simulink model "VSD_Motor_20kW"  (Simulink 9.3)
settings: Solver=ode23t  StartTime=0.0  StopTime=2  FixedStep=1e-5  MaxStep=1e-5  MinStep=1e-7  RelTol=1e-6  AbsTol=1e-6  EnableMultiTasking=on
libraries: powerlib x24, powerlib_extras x6, simulink x2
(part 1 of 2)
settings Model: Creator=Jiang  LastModifiedBy=Dominion
settings SolverCC: AutoScaleAbsTol=off
settings DataIOCC: LimitDataPoints=on
settings OptimizationCC: ExpressionDepthLimit=2147483647  InitFltsAndDblsToZero=on
settings DebuggingCC: SaveWithParameterizedLinksMsg=none  SignalResolutionControl=TryResolveAllWithWarning  SolverPrmCheckMsg=warning  MultiTaskDSMMsg=warning  MultiTaskCondExecSysMsg=none  StateNameClashWarn=warning
settings SFSimCC: SimUseLocalCustomCode=on
settings RTWCC: RTWUseLocalCustomCode=on
settings GRTTargetCC: TargetFcnLib=ansi_tfl_tmw.mat
settings ConfigComp: CovExternalEMLEnable=on

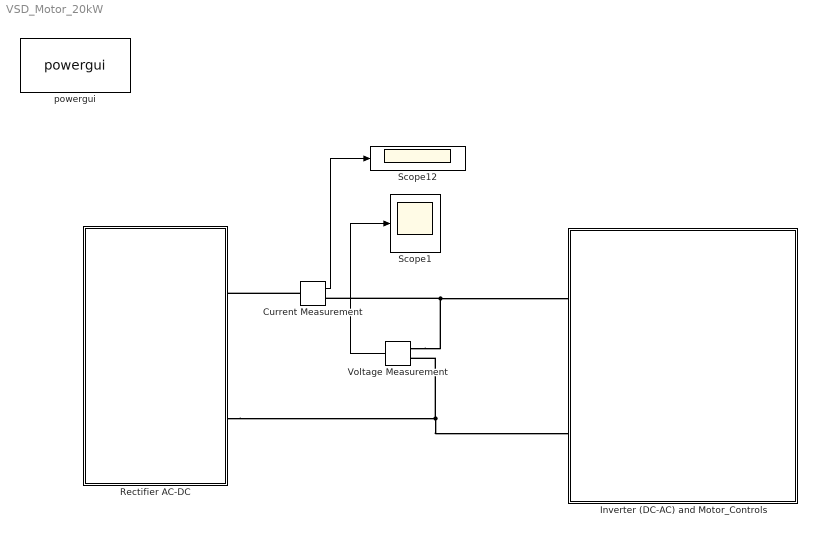
== system VSD_Motor_20kW ==
  Current Measurement : powerlib/Measurements/Current Measurement  PhasorSimulation=off  OutputType=Complex  PSBequivalent=0
      settings: SourceProductName=Simscape Electrical
  Inverter (DC-AC) and Motor_Controls : Subsystem
  Rectifier AC-DC : Subsystem
  Scope1 : Scope
  Scope12 : Scope
  Voltage Measurement : powerlib/Measurements/Voltage Measurement  PhasorSimulation=off  OutputType=Complex  PSBequivalent=0
      settings: SourceProductName=Simscape Electrical
  powergui : powerlib/powergui  SimulationMode=Discrete  SampleTime=2e-6  frequency=60  Iterations=50  frequencyindice=0  Pbase=100e6  ErrMax=1e-4  UnitsV=kV  UnitsW=MW  buscounter=0  FunctionMessages=off  echomessages=off  EnableUseOfTLC=off  CurrentSourceSwitches=off  DisableSnubberDevices=off  DisableRonSwitches=off  DisableVfSwitches=off  DisplayEquations=off  AutomaticDiscreteSolvers=off  SolverType=Tustin/Backward Euler (TBE)  Interpol=off  ExternalGateDelay=off  methode=off  Ts=0  x0status=blocks  SPID=off  SwTol=0  HookPort=off  NonlinearTolerance=0  nMaxIteration=15  ContinueOnMaxIteration=off  RestoreLinks=warning  ResistiveCurrentMeasurement=off  Frange=[0:2:500]  Ylog=off  Xlog=on  ShowGrid=off  save=off  variable=ZData  structure=0  ZoomFFT=on  StartTime=0.0  cycles=1  DisplayStyle=1  fundamental=60  FreqAxis=off  MaxFrequency=1000  frequencyindicesteady=1  RmsSteady=1  display=off
      settings: SourceProductName=Simscape Electrical
  wires:
  Voltage Measurement/1 -> Scope1/1
  Current Measurement/1 -> Scope12/1
  connections:
  Current Measurement/LConn1 -- Rectifier AC-DC/RConn1
  Voltage Measurement/LConn1 -- Current Measurement/RConn1 -- Inverter (DC-AC) and Motor_Controls/LConn1
  Rectifier AC-DC/RConn2 -- Voltage Measurement/LConn2 -- Inverter (DC-AC) and Motor_Controls/LConn2

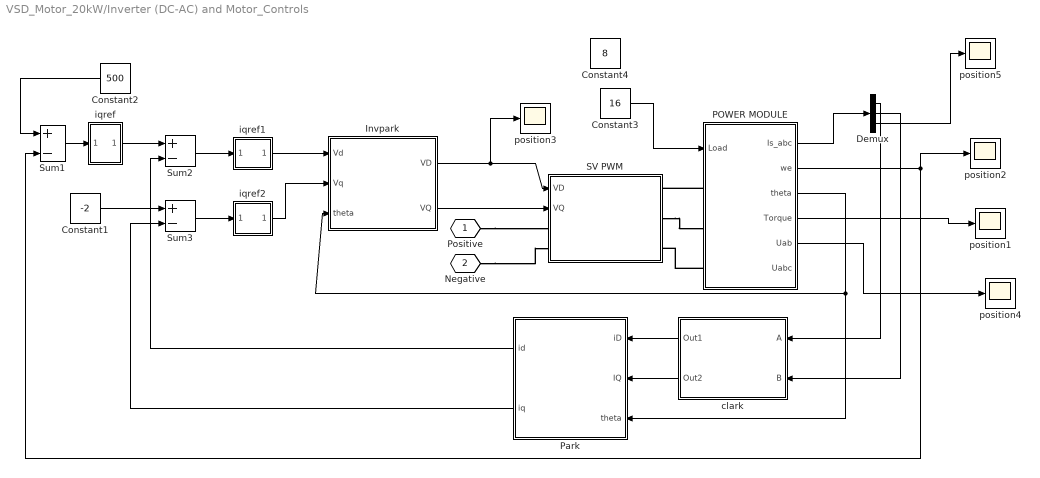
== system VSD_Motor_20kW/Inverter (DC-AC) and Motor_Controls ==
  Constant1 : Constant  Value=-2
  Constant2 : Constant  Value=500
  Constant3 : Constant  Value=16
  Constant4 : Constant  Value=8
  Demux : Demux  Outputs=3
  Invpark : Subsystem
  POWER MODULE : Subsystem
  Park : Subsystem
  SV PWM : Subsystem
  Sum1 : Sum  Inputs=+-  SaturateOnIntegerOverflow=on  InputSameDT=on  OutDataTypeStr=Inherit: Same as first input
  Sum2 : Sum  Inputs=+-  SaturateOnIntegerOverflow=on  InputSameDT=on  OutDataTypeStr=Inherit: Same as first input
  Sum3 : Sum  Inputs=+-  SaturateOnIntegerOverflow=on  InputSameDT=on  OutDataTypeStr=Inherit: Same as first input
  clark : Subsystem
  iqref : Subsystem  mask(PI Controller){I=20, P=0.2, sat=[-30,30]}
      mask prompts: I "Integral"; P "Proportional:"; sat "Minimum and maximum outputs:"
      mask init:
      | min=sat(1);max=sat(2);
      mask Display: disp('PI')
  iqref1 : Subsystem  mask(PI Controller){I=100, P=30, sat=[-400,400]}
      mask prompts: I "Integral"; P "Proportional:"; sat "Minimum and maximum outputs:"
      mask init:
      | min=sat(1);max=sat(2);
      mask Display: disp('PI')
  iqref2 : Subsystem  mask(PI Controller){I=100, P=30, sat=[-400,400]}
      mask prompts: I "Integral"; P "Proportional:"; sat "Minimum and maximum outputs:"
      mask init:
      | min=sat(1);max=sat(2);
      mask Display: disp('PI')
  position{1..5} (5 alike) : Scope
  Positive : PMIOPort  Tag=PMCPort  Side=Left
  Negative : PMIOPort  Tag=PMCPort  Port=2  Side=Left
  wires:
  Invpark/1(VD) -> SV PWM/1(VD), position3/1
  Invpark/2(VQ) -> SV PWM/2(VQ)
  Constant3/1 -> POWER MODULE/1(Load)
  POWER MODULE/1(Is_abc) -> Demux/1
  Demux/3 -> position5/1
  POWER MODULE/4(Torque) -> position1/1
  POWER MODULE/2(we) -> position2/1, Sum1/2
  Demux/1 -> clark/1(A)
  Demux/2 -> clark/2(B)
  clark/1(Out1) -> Park/1(iD)
  clark/2(Out2) -> Park/2(IQ)
  POWER MODULE/3(theta) -> Invpark/3(theta), Park/3(theta)
  Sum2/1 -> iqref1/1(In_1)
  Sum3/1 -> iqref2/1(In_1)
  Sum1/1 -> iqref/1(In_1)
  iqref2/1(Out_1) -> Invpark/2(Vq)
  iqref1/1(Out_1) -> Invpark/1(Vd)
  iqref/1(Out_1) -> Sum2/1
  Constant1/1 -> Sum3/1
  Constant2/1 -> Sum1/1
  Park/2(iq) -> Sum3/2
  Park/1(id) -> Sum2/2
  POWER MODULE/5(Uab) -> position4/1
  connections:
  POWER MODULE/LConn1 -- SV PWM/RConn1
  SV PWM/RConn2 -- POWER MODULE/LConn2
  POWER MODULE/LConn3 -- SV PWM/RConn3
  Negative/RConn1 -- SV PWM/LConn2
  Positive/RConn1 -- SV PWM/LConn1

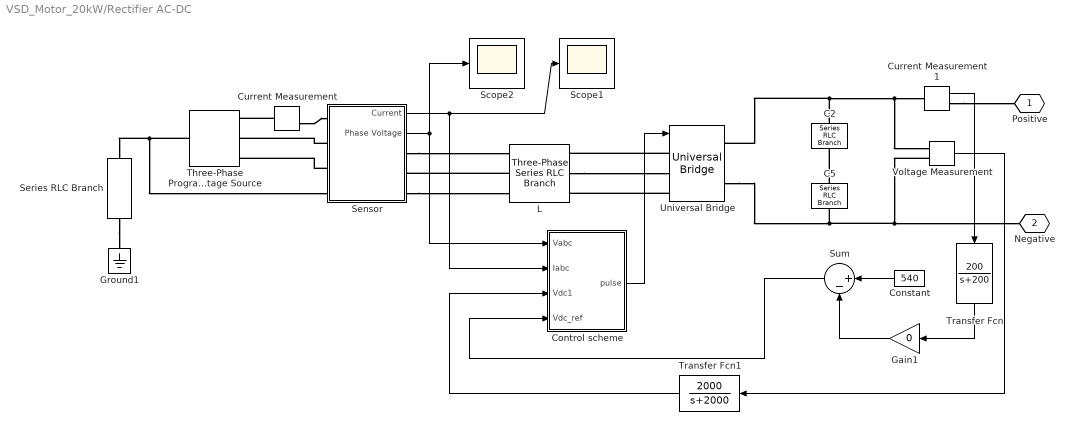
== system VSD_Motor_20kW/Rectifier AC-DC ==
  C2 : powerlib/Elements/Series RLC Branch  LConnTagsString=__new0  RConnTagsString=__new0  BranchType=C  Resistance=1.0  Inductance=1.0  SetiL0=off  InitialCurrent=0  Capacitance=6e-04  Setx0=on  InitialVoltage=100  Measurements=None
      settings: SourceProductName=Simscape Electrical
  C5 : powerlib/Elements/Series RLC Branch  LConnTagsString=__new0  RConnTagsString=__new0  BranchType=C  Resistance=1.0  Inductance=1.0  SetiL0=off  InitialCurrent=0  Capacitance=6e-04  Setx0=on  InitialVoltage=100  Measurements=None
      settings: SourceProductName=Simscape Electrical
  Constant : Constant  Value=540
  Control scheme : Subsystem
  Current Measurement : powerlib/Measurements/Current Measurement  PhasorSimulation=off  OutputType=Complex  PSBequivalent=0
      settings: SourceProductName=Simscape Electrical
  Current Measurement1 : powerlib/Measurements/Current Measurement  PhasorSimulation=off  OutputType=Complex  PSBequivalent=0
      settings: SourceProductName=Simscape Electrical
  Gain1 : Gain  Gain=0
  Ground1 : powerlib/Elements/Ground  LConnTagsString=a
      settings: SourceProductName=Simscape Electrical
  L : powerlib/Elements/Three-Phase Series RLC Branch  LConnTagsString=A|B|C  RConnTagsString=A|B|C  BranchType=RL  Resistance=0.0001  Inductance=3.5e-3  Capacitance=1.0  Measurements=None
      settings: SourceProductName=Simscape Electrical
  Scope1 : Scope
  Scope2 : Scope
  Sensor : Subsystem
  Series RLC Branch : powerlib/Elements/Series RLC Branch  LConnTagsString=__new0  RConnTagsString=__new0  BranchType=R  Resistance=1e5  Inductance=1e-3  SetiL0=off  InitialCurrent=0  Capacitance=1e-6  Setx0=off  InitialVoltage=0  Measurements=None
      settings: SourceProductName=Simscape Electrical
  Sum : Sum  Inputs=|+-  SaturateOnIntegerOverflow=on  InputSameDT=on  OutDataTypeStr=Inherit: Same as first input
  Three-Phase Programmable Voltage Source : powerlib/Electrical Sources/Three-Phase Programmable Voltage Source  PositiveSequence=[400 0 60]  VariationEntity=None  VariationType=Step  VariationTypeAlt=Step  VariationStep=0.5  VariationRate=10  VariationMagnitude=0.3  VariationFrequency=2  VariationTiming=[1 2]  VariationPhaseA=off  Amplitudes=[1 0.8 1.2 1.0]  TimeValues=[0 0.1 0.15 0.2]  HarmonicGeneration=off  HarmonicA=[3 0.2 -25 0]  HarmonicB=[2 0.15 35 2]  Timing="[0.05  3]"  BusType=swing  Pref=0  Qref=0  Qmin=-inf  Qmax=inf
      settings: SourceProductName=Simscape Electrical
  Transfer Fcn : TransferFcn  Numerator=[200]  Denominator=[1 200]
  Transfer Fcn1 : TransferFcn  Numerator=[2000]  Denominator=[1 2000]
  Universal Bridge : powerlib/Power Electronics/Universal Bridge  Arms=3  SnubberResistance=50000  SnubberCapacitance=1e-8  Device=MOSFET / Diodes  Ron=0.2e-4  Lon=0  ForwardVoltages="[  2 1  ]"  ForwardVoltage=0  GTOparameters=[ 10e-6 , 20e-6 ]  IGBTparameters=[ 1e-6 , 2e-6 ]  Measurements=None  Measurements_2=None  converterType=Rectifier
      settings: SourceProductName=Simscape Electrical
  Voltage Measurement : powerlib/Measurements/Voltage Measurement  PhasorSimulation=off  OutputType=Complex  PSBequivalent=0
      settings: SourceProductName=Simscape Electrical
  Positive : PMIOPort  Tag=PMCPort  Side=Right
  Negative : PMIOPort  Tag=PMCPort  Port=2  Side=Right
  wires:
  Voltage Measurement/1 -> Transfer Fcn1/1
  Control scheme/1(pulse) -> Universal Bridge/1
  Constant/1 -> Sum/1
  Gain1/1 -> Sum/2
  Sum/1 -> Control scheme/4(Vdc_ref)
  Sensor/1(Current) -> Control scheme/2(Iabc), Scope1/1
  Sensor/2(Phase Voltage) -> Control scheme/1(Vabc), Scope2/1
  Transfer Fcn/1 -> Gain1/1
  Transfer Fcn1/1 -> Control scheme/3(Vdc1)
  Current Measurement1/1 -> Transfer Fcn/1
  connections:
  L/LConn2 -- Sensor/RConn2
  Universal Bridge/LConn1 -- L/RConn1
  L/RConn2 -- Universal Bridge/LConn2
  Current Measurement/LConn1 -- Three-Phase Programmable Voltage Source/RConn1
  Sensor/RConn1 -- L/LConn1
  Universal Bridge/LConn3 -- L/RConn3
  Sensor/RConn3 -- L/LConn3
  Current Measurement/RConn1 -- Sensor/LConn1
  Sensor/LConn2 -- Three-Phase Programmable Voltage Source/RConn2
  Sensor/LConn3 -- Three-Phase Programmable Voltage Source/RConn3
  Universal Bridge/RConn1 -- C2/LConn1 -- Voltage Measurement/LConn1 -- Current Measurement1/LConn1
  Voltage Measurement/LConn2 -- Negative/RConn1 -- Universal Bridge/RConn2 -- C5/RConn1
  C5/LConn1 -- C2/RConn1
  Three-Phase Programmable Voltage Source/LConn1 -- Sensor/LConn4 -- Series RLC Branch/LConn1
  Current Measurement1/RConn1 -- Positive/RConn1
  Series RLC Branch/RConn1 -- Ground1/LConn1

== system VSD_Motor_20kW/Inverter (DC-AC) and Motor_Controls/Invpark ==
  Vd : Inport
  Vq : Inport  Port=2
  theta : Inport  Port=3
  Product{,1..3} (4 alike) : Product  RndMeth=Zero
  Sum2 : Sum  Inputs=|-+
  Sum3 : Sum  Inputs=|++
  Trigonometric Function : Trigonometry
  Trigonometric Function1 : Trigonometry  Operator=cos
  VD : Outport
  VQ : Outport  Port=2
  wires:
  Trigonometric Function1/1 -> Product/2, Product3/2
  Trigonometric Function/1 -> Product1/2, Product2/2
  Product1/1 -> Sum2/1
  Product/1 -> Sum2/2
  Sum2/1 -> VD/1
  Product2/1 -> Sum3/2
  Product3/1 -> Sum3/1
  Sum3/1 -> VQ/1
  theta/1 -> Trigonometric Function/1, Trigonometric Function1/1
  Vd/1 -> Product/1, Product2/1
  Vq/1 -> Product1/1, Product3/1

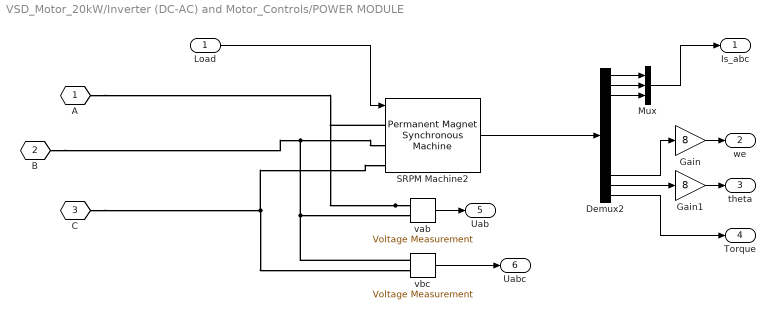
== system VSD_Motor_20kW/Inverter (DC-AC) and Motor_Controls/POWER MODULE ==
  Load : Inport
  Demux2 : Demux  Outputs=13
  Gain : Gain  Gain=8
  Gain1 : Gain  Gain=8
  Mux : Mux  Inputs=3
  SRPM Machine2 : powerlib/Machines/Permanent Magnet Synchronous Machine  NbPhases=3  FluxDistribution=Sinusoidal  RotorType=Round  MechanicalLoad=Torque Tm  PresetModel=No  ShowDetailedParameters=on  MeasurementBus=off  Resistance=0.7  Inductance=8.5e-3  dqInductances=[0.01 0.01]  La=0.000395  MachineConstant=Flux linkage established by magnets (V.s)  Flux=0.1  VoltageCst=145.1039  TorqueCst=1.2  Flat=120  Mechanical="[ 2e-4, 0,  8 ]"  PolePairs=4  InitialConditions=[0,0, 0,0]  InitialConditions5ph=[0 0 0 0 0 0]  TsPowergui=0  TsBlock=-1  RefAngle=90 degrees behind phase A axis (modified Park)
      settings: AttributesFormatString=\n
  vab : powerlib/Measurements/Voltage Measurement  Tag=PoWeRsYsTeMmEaSuReMeNt  PhasorSimulation=off  OutputType=Magnitude  PSBequivalent=0
      settings: SourceProductName=Simscape Electrical
  vbc : powerlib/Measurements/Voltage Measurement  Tag=PoWeRsYsTeMmEaSuReMeNt  PhasorSimulation=off  OutputType=Magnitude  PSBequivalent=0
      settings: SourceProductName=Simscape Electrical
  A : PMIOPort  Tag=PMCPort  Side=Left
  B : PMIOPort  Tag=PMCPort  Port=2  Side=Left
  C : PMIOPort  Tag=PMCPort  Port=3  Side=Left
  Is_abc : Outport
  we : Outport  Port=2
  theta : Outport  Port=3
  Torque : Outport  Port=4
  Uab : Outport  Port=5
  Uabc : Outport  Port=6
  wires:
  SRPM Machine2/1 -> Demux2/1
  Load/1 -> SRPM Machine2/1
  Demux2/1 -> Mux/1
  Demux2/2 -> Mux/2
  Demux2/3 -> Mux/3
  Mux/1 -> Is_abc/1
  Demux2/11 -> Gain/1
  Demux2/12 -> Gain1/1
  Demux2/13 -> Torque/1
  vab/1 -> Uab/1
  Gain/1 -> we/1
  Gain1/1 -> theta/1
  vbc/1 -> Uabc/1
  connections:
  vab/LConn1 -- A/RConn1 -- SRPM Machine2/LConn1
  vbc/LConn1 -- vab/LConn2 -- B/RConn1 -- SRPM Machine2/LConn2
  C/RConn1 -- SRPM Machine2/LConn3 -- vbc/LConn2

== system VSD_Motor_20kW/Inverter (DC-AC) and Motor_Controls/Park ==
  iD : Inport
  IQ : Inport  Port=2
  theta : Inport  Port=3
  Product{,1..3} (4 alike) : Product  RndMeth=Zero
  Sum1 : Sum  Inputs=|++
  Sum2 : Sum  Inputs=|+-
  Trigonometric Function : Trigonometry
  Trigonometric Function1 : Trigonometry  Operator=cos
  id : Outport
  iq : Outport  Port=2
  wires:
  theta/1 -> Trigonometric Function1/1, Trigonometric Function/1
  Trigonometric Function1/1 -> Product/2, Product3/2
  Trigonometric Function/1 -> Product1/2, Product2/2
  IQ/1 -> Product1/1, Product3/1
  iD/1 -> Product/1, Product2/1
  Product1/1 -> Sum1/1
  Product/1 -> Sum1/2
  Sum1/1 -> id/1
  Product2/1 -> Sum2/2
  Product3/1 -> Sum2/1
  Sum2/1 -> iq/1

== system VSD_Motor_20kW/Inverter (DC-AC) and Motor_Controls/SV PWM ==
  VD : Inport
  VQ : Inport  Port=2
  SVPWM : Subsystem  mask(SVPWM){Ts=1/2e4}
      mask prompts: Ts "switching frequency"
      mask help: two-level svpwm generator
  Universal Bridge1 : powerlib/Power Electronics/Universal Bridge  Arms=3  SnubberResistance=1e5  SnubberCapacitance=inf  Device=MOSFET / Diodes  Ron=1e-3  Lon=0  ForwardVoltages="[  0  0  ]"  ForwardVoltage=0  GTOparameters=[ 10e-6 , 20e-6 ]  IGBTparameters=[ 1e-6 , 2e-6 ]  Measurements=None  Measurements_2=None  converterType=Rectifier
      settings: SourceProductName=Simscape Electrical
  vdc : powerlib/Measurements/Voltage Measurement  Tag=PoWeRsYsTeMmEaSuReMeNt  PhasorSimulation=off  OutputType=Magnitude  PSBequivalent=0
      settings: SourceProductName=Simscape Electrical
  Positive : PMIOPort  Tag=PMCPort  Side=Left
  negative : PMIOPort  Tag=PMCPort  Port=2  Side=Left
  A : PMIOPort  Tag=PMCPort  Port=3  Side=Right
  B : PMIOPort  Tag=PMCPort  Port=4  Side=Right
  C : PMIOPort  Tag=PMCPort  Port=5  Side=Right
  wires:
  VD/1 -> SVPWM/2(Valf)
  VQ/1 -> SVPWM/3(Vbeta)
  SVPWM/1(Out1) -> Universal Bridge1/1
  vdc/1 -> SVPWM/1(Udc)
  connections:
  Positive/RConn1 -- Universal Bridge1/RConn1 -- vdc/LConn1
  negative/RConn1 -- Universal Bridge1/RConn2 -- vdc/LConn2
  C/RConn1 -- Universal Bridge1/LConn3
  B/RConn1 -- Universal Bridge1/LConn2
  A/RConn1 -- Universal Bridge1/LConn1

== system VSD_Motor_20kW/Inverter (DC-AC) and Motor_Controls/clark ==
  A : Inport
  B : Inport  Port=2
  Gain : Gain  Gain=3/2
  Gain1 : Gain  Gain=2/sqrt(3)
  Gain2 : Gain  Gain=1/sqrt(3)
  Gain3 : Gain  Gain=3/2
  Gain4 : Gain  Gain=sqrt(2/3)
  Gain5 : Gain  Gain=sqrt(2/3)
  Sum1 : Sum  Inputs=|++
  Out1 : Outport
  Out2 : Outport  Port=2
  wires:
  A/1 -> Gain2/1, Gain3/1
  B/1 -> Gain1/1
  Gain2/1 -> Sum1/1
  Gain1/1 -> Sum1/2
  Sum1/1 -> Gain/1
  Gain3/1 -> Gain4/1
  Gain/1 -> Gain5/1
  Gain4/1 -> Out1/1
  Gain5/1 -> Out2/1

== system VSD_Motor_20kW/Inverter (DC-AC) and Motor_Controls/iqref ==
  In_1 : Inport
  Integral : TransferFcn  Numerator=[I]  Denominator=[1 0]
  Proportional : Gain  Gain=P  SaturateOnIntegerOverflow=on  OutDataTypeStr=Inherit: Same as input  ParamDataTypeStr=Inherit: Same as input
  Saturation : Saturate  UpperLimit=max  LowerLimit=min
  Sum : Sum  SaturateOnIntegerOverflow=on  InputSameDT=on  OutDataTypeStr=Inherit: Same as first input
  Out_1 : Outport  InitialOutput=0
  wires:
  Integral/1 -> Sum/2
  In_1/1 -> Integral/1, Proportional/1
  Proportional/1 -> Sum/1
  Sum/1 -> Saturation/1
  Saturation/1 -> Out_1/1

== system VSD_Motor_20kW/Inverter (DC-AC) and Motor_Controls/iqref1 ==
  In_1 : Inport
  Integral : TransferFcn  Numerator=[I]  Denominator=[1 0]
  Proportional : Gain  Gain=P  SaturateOnIntegerOverflow=on  OutDataTypeStr=Inherit: Same as input  ParamDataTypeStr=Inherit: Same as input
  Saturation : Saturate  UpperLimit=max  LowerLimit=min
  Sum : Sum  SaturateOnIntegerOverflow=on  InputSameDT=on  OutDataTypeStr=Inherit: Same as first input
  Out_1 : Outport  InitialOutput=0
  wires:
  Integral/1 -> Sum/2
  In_1/1 -> Integral/1, Proportional/1
  Proportional/1 -> Sum/1
  Sum/1 -> Saturation/1
  Saturation/1 -> Out_1/1

== system VSD_Motor_20kW/Inverter (DC-AC) and Motor_Controls/iqref2 ==
  In_1 : Inport
  Integral : TransferFcn  Numerator=[I]  Denominator=[1 0]
  Proportional : Gain  Gain=P  SaturateOnIntegerOverflow=on  OutDataTypeStr=Inherit: Same as input  ParamDataTypeStr=Inherit: Same as input
  Saturation : Saturate  UpperLimit=max  LowerLimit=min
  Sum : Sum  SaturateOnIntegerOverflow=on  InputSameDT=on  OutDataTypeStr=Inherit: Same as first input
  Out_1 : Outport  InitialOutput=0
  wires:
  Integral/1 -> Sum/2
  In_1/1 -> Integral/1, Proportional/1
  Proportional/1 -> Sum/1
  Sum/1 -> Saturation/1
  Saturation/1 -> Out_1/1

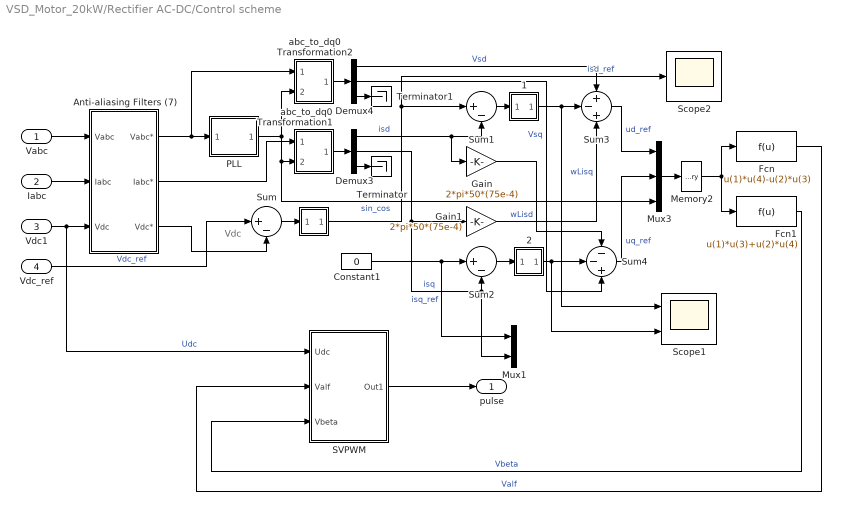
== system VSD_Motor_20kW/Rectifier AC-DC/Control scheme ==
  note: Vdc
  Vabc : Inport  PortDimensions=3
  Iabc : Inport  Port=2  PortDimensions=3
  Vdc1 : Inport  Port=3  PortDimensions=1
  Vdc_ref : Inport  Port=4  PortDimensions=1
  " " : Subsystem  mask(PI Controller){I=100, P=0.07, sat=[-200,200]}
      mask prompts: I "Integral"; P "Proportional:"; sat "Minimum and maximum outputs:"
      mask init:
      | min=sat(1);max=sat(2);
      mask Display: disp('PI')
  " 1" : Subsystem  mask(PI Controller){I=100, P=20, sat=[-1000*1.2, 1000*1.2]}
      mask prompts: I "Integral"; P "Proportional:"; sat "Minimum and maximum outputs:"
      mask init:
      | min=sat(1);max=sat(2);
      mask Display: disp('PI')
  " 2" : Subsystem  mask(PI Controller){I=100, P=20, sat=[-1000*1.2, 1000*1.2]}
      mask prompts: I "Integral"; P "Proportional:"; sat "Minimum and maximum outputs:"
      mask init:
      | min=sat(1);max=sat(2);
      mask Display: disp('PI')
  Anti-aliasing Filters (7) : Subsystem  mask(Anti-aliasing (2nd order lowpass)){Fc=750, Ts=-1}
      mask prompts: Fc "Cut-off frequency (Hz):"; Ts "Sample time:"
  Constant1 : Constant  Value=0
  Demux3 : Demux  Outputs=3
  Demux4 : Demux  Outputs=3
  Fcn : Fcn  Expr=u(1)*u(4)-u(2)*u(3)
  Fcn1 : Fcn  Expr=u(1)*u(3)+u(2)*u(4)
  Gain : Gain  Gain=2*pi*50*(75e-4)
  Gain1 : Gain  Gain=2*pi*50*(75e-4)
  Memory2 : Memory
  Mux1 : Mux  Inputs=2
  Mux3 : Mux  Inputs=3
  PLL : Subsystem
  SVPWM : Subsystem  mask(SVPWM){Ts=1/5e3}
      mask prompts: Ts "switching frequency"
      mask help: two-level svpwm generator
  Scope1 : Scope  NumInputPorts=2
  Scope2 : Scope
  Sum : Sum  Inputs=|+-  SaturateOnIntegerOverflow=on  InputSameDT=on  OutDataTypeStr=Inherit: Same as first input
  Sum1 : Sum  Inputs=|+-  SaturateOnIntegerOverflow=on  InputSameDT=on  OutDataTypeStr=Inherit: Same as first input
  Sum2 : Sum  Inputs=|+-  SaturateOnIntegerOverflow=on  InputSameDT=on  OutDataTypeStr=Inherit: Same as first input
  Sum3 : Sum  Inputs=+-+  SaturateOnIntegerOverflow=on  InputSameDT=on  OutDataTypeStr=Inherit: Same as first input
  Sum4 : Sum  Inputs=--+  SaturateOnIntegerOverflow=on  InputSameDT=on  OutDataTypeStr=Inherit: Same as first input
  Terminator : Terminator
  Terminator1 : Terminator
  abc_to_dq0 Transformation1 : Subsystem  mask(abc to dq0 Transformation){}
      mask help:
      | This block performs the  abc to dq0 transformation on a set of three-phase signals. It computes the direct axis Vd, quadratic axis Vq, and zero sequence V0 quantities in a two axis rotating reference frame according to the following transformation:
      |
      | Vd = 2/3*[Va*sin(wt)  + Vb*sin(wt-2pi/3)  +  Vc*sin(wt+2pi/3)]
      | Vq = 2/3*[Va*cos(wt) + Vb*cos(wt-2pi/3) + Vc*cos(wt+2pi/3)]
      | V0 = 1/3*[Va +  Vb  +  Vc ]
      |
      | where w=  rotation speed (rad/s) of the rotating frame.
      |
      | This transformation is commonly used in three-phase electric machine models where it is known as the Park transformation.
      mask Help: web(psbhelp);
  abc_to_dq0 Transformation2 : Subsystem  mask(abc to dq0 Transformation){}
      mask help:
      | This block performs the  abc to dq0 transformation on a set of three-phase signals. It computes the direct axis Vd, quadratic axis Vq, and zero sequence V0 quantities in a two axis rotating reference frame according to the following transformation:
      |
      | Vd = 2/3*[Va*sin(wt)  + Vb*sin(wt-2pi/3)  +  Vc*sin(wt+2pi/3)]
      | Vq = 2/3*[Va*cos(wt) + Vb*cos(wt-2pi/3) + Vc*cos(wt+2pi/3)]
      | V0 = 1/3*[Va +  Vb  +  Vc ]
      |
      | where w=  rotation speed (rad/s) of the rotating frame.
      |
      | This transformation is commonly used in three-phase electric machine models where it is known as the Park transformation.
      mask Help: web(psbhelp);
  pulse : Outport
  wires:
  Vdc1/1 -> Anti-aliasing Filters (7)/3("Vdc "), SVPWM/1(Udc)  "Udc"
  Iabc/1 -> Anti-aliasing Filters (7)/2("Iabc ")
  Vabc/1 -> Anti-aliasing Filters (7)/1(Vabc)
  Vdc_ref/1 -> Sum/1  "Vdc_ref"
  abc_to_dq0 Transformation1/1(dq0) -> Demux3/1
  Anti-aliasing Filters (7)/1(" Vabc*") -> PLL/1(Vabc), abc_to_dq0 Transformation2/1(abc)
  Anti-aliasing Filters (7)/3(" Vdc*") -> Sum/2
  " "/1(Out_1) -> Sum1/1, Scope2/1  "isd_ref"
  Sum2/1 -> " 2"/1(In_1)
  Anti-aliasing Filters (7)/2(Iabc*) -> abc_to_dq0 Transformation1/1(abc)
  PLL/1(sin-cos) -> abc_to_dq0 Transformation2/2(sin_cos), Mux3/3, abc_to_dq0 Transformation1/2(sin_cos)  "sin_cos"
  Constant1/1 -> Sum2/1, Mux1/1  "isq_ref"
  Demux3/1 -> Sum1/2, Gain/1  "isd"
  Demux3/2 -> Gain1/1, Sum2/2, Mux1/2  "isq"
  Demux3/3 -> Terminator/1
  Sum1/1 -> " 1"/1(In_1)
  Demux4/3 -> Terminator1/1
  abc_to_dq0 Transformation2/1(dq0) -> Demux4/1
  " 1"/1(Out_1) -> Sum3/2, Scope1/1
  " 2"/1(Out_1) -> Sum4/2, Scope1/2
  Sum3/1 -> Mux3/1  "ud_ref"
  Sum4/1 -> Mux3/2  "uq_ref"
  Mux3/1 -> Memory2/1
  Fcn/1 -> SVPWM/2(Valf)  "Valf"
  Fcn1/1 -> SVPWM/3(Vbeta)  "Vbeta"
  SVPWM/1(Out1) -> pulse/1
  Demux4/1 -> Sum3/1  "Vsd"
  Demux4/2 -> Sum4/3  "Vsq"
  Sum/1 -> " "/1(In_1)
  Memory2/1 -> Fcn/1, Fcn1/1
  Gain1/1 -> Sum3/3  "wLisq"
  Gain/1 -> Sum4/1  "wLisd"

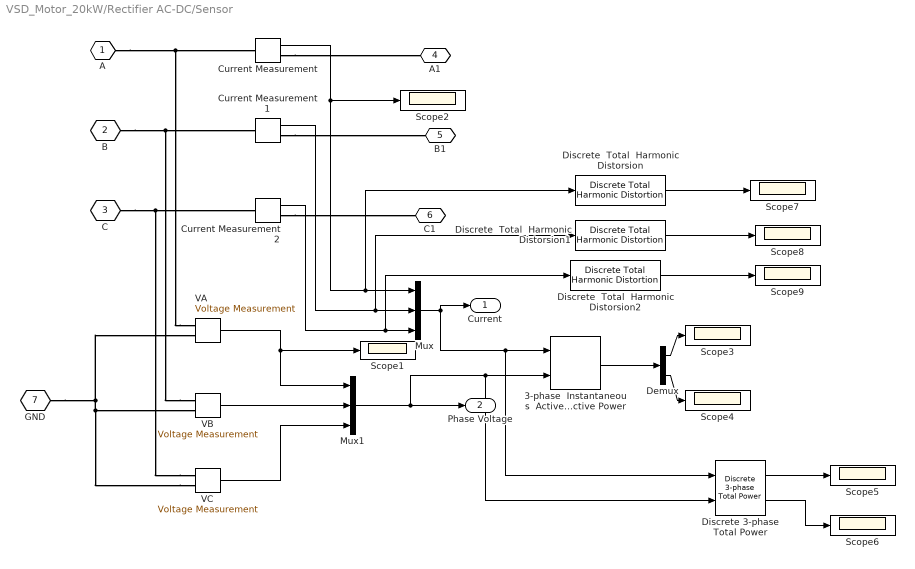
== system VSD_Motor_20kW/Rectifier AC-DC/Sensor ==
  3-phase  Instantaneous  Active & Reactive Power : powerlib_extras/Measurements/3-phase  Instantaneous  Active & Reactive Power
      settings: SourceProductName=Simscape Electrical  SourceProductBaseCode=PS
  Current Measurement : powerlib/Measurements/Current Measurement  PhasorSimulation=off  OutputType=Complex  PSBequivalent=0
      settings: SourceProductName=Simscape Electrical
  Current Measurement1 : powerlib/Measurements/Current Measurement  PhasorSimulation=off  OutputType=Complex  PSBequivalent=0
      settings: SourceProductName=Simscape Electrical
  Current Measurement2 : powerlib/Measurements/Current Measurement  PhasorSimulation=off  OutputType=Complex  PSBequivalent=0
      settings: SourceProductName=Simscape Electrical
  Demux : Demux  Outputs=2
  Discrete  Total  Harmonic Distorsion : powerlib_extras/Discrete Measurements/Discrete Total Harmonic Distortion  Freq=50  Ts=5e-6
      settings: SourceProductName=Simscape Electrical  SourceProductBaseCode=PS
  Discrete  Total  Harmonic Distorsion1 : powerlib_extras/Discrete Measurements/Discrete Total Harmonic Distortion  Freq=50  Ts=5e-6
      settings: SourceProductName=Simscape Electrical  SourceProductBaseCode=PS
  Discrete  Total  Harmonic Distorsion2 : powerlib_extras/Discrete Measurements/Discrete Total Harmonic Distortion  Freq=50  Ts=5e-6
      settings: SourceProductName=Simscape Electrical  SourceProductBaseCode=PS
  Discrete 3-phase Total Power : powerlib_extras/Discrete Measurements/Discrete 3-phase Total Power  Freq=50  Par_Vinit=[0 0]  Par_Iinit=[0 0]  Ts=5e-6
      settings: SourceProductName=Simscape Electrical  SourceProductBaseCode=PS
  Mux : Mux  Inputs=3
  Mux1 : Mux  Inputs=3
  Scope{1..9} (9 alike) : Scope
  VA : powerlib/Measurements/Voltage Measurement  PhasorSimulation=off  OutputType=Complex  PSBequivalent=0
      settings: SourceProductName=Simscape Electrical
  VB : powerlib/Measurements/Voltage Measurement  PhasorSimulation=off  OutputType=Complex  PSBequivalent=0
      settings: SourceProductName=Simscape Electrical
  VC : powerlib/Measurements/Voltage Measurement  PhasorSimulation=off  OutputType=Complex  PSBequivalent=0
      settings: SourceProductName=Simscape Electrical
  A : PMIOPort  Side=Left
  B : PMIOPort  Port=2  Side=Left
  C : PMIOPort  Port=3  Side=Left
  A1 : PMIOPort  Port=4  Side=Right
  B1 : PMIOPort  Port=5  Side=Right
  C1 : PMIOPort  Port=6  Side=Right
  GND : PMIOPort  Port=7  Side=Left
  Current : Outport
  Phase Voltage : Outport  Port=2
  wires:
  Current Measurement/1 -> Scope2/1, Mux/1, Discrete  Total  Harmonic Distorsion/1
  Current Measurement1/1 -> Mux/2, Discrete  Total  Harmonic Distorsion1/1
  Current Measurement2/1 -> Mux/3, Discrete  Total  Harmonic Distorsion2/1
  Mux/1 -> Current/1, 3-phase  Instantaneous  Active & Reactive Power/1, Discrete 3-phase Total Power/1
  Mux1/1 -> Phase Voltage/1, 3-phase  Instantaneous  Active & Reactive Power/2, Discrete 3-phase Total Power/2
  VA/1 -> Mux1/1, Scope1/1
  VB/1 -> Mux1/2
  VC/1 -> Mux1/3
  3-phase  Instantaneous  Active & Reactive Power/1 -> Demux/1
  Demux/1 -> Scope3/1
  Demux/2 -> Scope4/1
  Discrete 3-phase Total Power/1 -> Scope5/1
  Discrete 3-phase Total Power/2 -> Scope6/1
  Discrete  Total  Harmonic Distorsion/1 -> Scope7/1
  Discrete  Total  Harmonic Distorsion1/1 -> Scope8/1
  Discrete  Total  Harmonic Distorsion2/1 -> Scope9/1
  connections:
  VA/LConn1 -- A/RConn1 -- Current Measurement/LConn1
  VB/LConn1 -- B/RConn1 -- Current Measurement1/LConn1
  VC/LConn1 -- C/RConn1 -- Current Measurement2/LConn1
  Current Measurement/RConn1 -- A1/RConn1
  Current Measurement1/RConn1 -- B1/RConn1
  Current Measurement2/RConn1 -- C1/RConn1
  VC/LConn2 -- GND/RConn1 -- VA/LConn2 -- VB/LConn2

== system VSD_Motor_20kW/Inverter (DC-AC) and Motor_Controls/SV PWM/SVPWM ==
  note: Subsystem1: calculate the work time of the vector
  note: sector calc: calculate the sector of the reference vector
  Udc : Inport
  Valf : Inport  Port=2
  Vbeta : Inport  Port=3
  Mux1 : Mux  Inputs=2
  Scope1 : Scope  NumInputPorts=2
  Scope2 : Scope
  Scope5 : Scope
  Scope7 : Scope
  T1 : Constant  Value=Ts
  pulse generater : Subsystem
  sector calc : Subsystem
  time calc : Subsystem
  time convert : Subsystem
  time convert1 : Subsystem
  time convert2 : Subsystem
  triangular : simulink/Sources/Repeating Sequence  rep_seq_t=[0 0.5 1]*Ts  rep_seq_y=[0 0.5 0]*Ts
  Out1 : Outport
  wires:
  Mux1/1 -> Scope5/1
  triangular/1 -> pulse generater/4(Tri), Mux1/1, Scope7/1
  time convert2/3(Tcm3) -> pulse generater/3(Tcm3)
  time convert2/2(Tcm2) -> pulse generater/2(Tcm2)
  time convert1/3(Tc) -> time convert2/3(Tc)
  time convert1/2(Tb) -> time convert2/2(Tb)
  time convert1/1(Ta) -> time convert2/1(Ta)
  time convert2/1(Tcm1) -> pulse generater/1(Tcm1), Mux1/2
  time convert/2(t2) -> time convert1/3(t2)
  time convert/1(t1) -> time convert1/2(t1)
  T1/1 -> time calc/2(In2), time convert1/1(Ts)
  sector calc/1(N) -> time convert/4(N), time convert2/4(N), Scope2/1
  time calc/3(Z) -> time convert/3(Z)
  time calc/2(Y) -> time convert/2(Y)
  time calc/1(X) -> time convert/1(X)
  Udc/1 -> time calc/1(In1)
  Vbeta/1 -> sector calc/2(ubeta), time calc/3(In3), Scope1/2
  Valf/1 -> sector calc/1(ualf), Scope1/1, time calc/4(In4)
  pulse generater/1(pulse) -> Out1/1

== system VSD_Motor_20kW/Rectifier AC-DC/Control scheme/  ==
  In_1 : Inport
  Integral : TransferFcn  Numerator=[I]  Denominator=[1 0]
  Proportional : Gain  Gain=P  SaturateOnIntegerOverflow=on  OutDataTypeStr=Inherit: Same as input  ParamDataTypeStr=Inherit: Same as input
  Saturation : Saturate  UpperLimit=max  LowerLimit=min
  Saturation1 : Saturate  UpperLimit=max  LowerLimit=min
  Sum : Sum  SaturateOnIntegerOverflow=on  InputSameDT=on  OutDataTypeStr=Inherit: Same as first input
  Out_1 : Outport  InitialOutput=0
  wires:
  Integral/1 -> Saturation1/1
  In_1/1 -> Integral/1, Proportional/1
  Proportional/1 -> Sum/1
  Sum/1 -> Saturation/1
  Saturation/1 -> Out_1/1
  Saturation1/1 -> Sum/2

== system VSD_Motor_20kW/Rectifier AC-DC/Control scheme/ 1 ==
  In_1 : Inport
  Integral : TransferFcn  Numerator=[I]  Denominator=[1 0]
  Proportional : Gain  Gain=P  SaturateOnIntegerOverflow=on  OutDataTypeStr=Inherit: Same as input  ParamDataTypeStr=Inherit: Same as input
  Saturation : Saturate  UpperLimit=max  LowerLimit=min
  Saturation1 : Saturate  UpperLimit=max  LowerLimit=min
  Sum : Sum  SaturateOnIntegerOverflow=on  InputSameDT=on  OutDataTypeStr=Inherit: Same as first input
  Out_1 : Outport  InitialOutput=0
  wires:
  Saturation1/1 -> Sum/2
  Saturation/1 -> Out_1/1
  Sum/1 -> Saturation/1
  Proportional/1 -> Sum/1
  In_1/1 -> Proportional/1, Integral/1
  Integral/1 -> Saturation1/1

== system VSD_Motor_20kW/Rectifier AC-DC/Control scheme/ 2 ==
  In_1 : Inport
  Integral : TransferFcn  Numerator=[I]  Denominator=[1 0]
  Proportional : Gain  Gain=P  SaturateOnIntegerOverflow=on  OutDataTypeStr=Inherit: Same as input  ParamDataTypeStr=Inherit: Same as input
  Saturation : Saturate  UpperLimit=max  LowerLimit=min
  Saturation1 : Saturate  UpperLimit=max  LowerLimit=min
  Sum : Sum  SaturateOnIntegerOverflow=on  InputSameDT=on  OutDataTypeStr=Inherit: Same as first input
  Out_1 : Outport  InitialOutput=0
  wires:
  Integral/1 -> Saturation1/1
  In_1/1 -> Integral/1, Proportional/1
  Proportional/1 -> Sum/1
  Sum/1 -> Saturation/1
  Saturation/1 -> Out_1/1
  Saturation1/1 -> Sum/2

== system VSD_Motor_20kW/Rectifier AC-DC/Control scheme/Anti-aliasing Filters (7) ==
  Vabc : Inport  PortDimensions=3
  "Iabc " : Inport  Port=2  PortDimensions=3
  "Vdc " : Inport  Port=3  PortDimensions=1
  2nd-Order Filter8 : powerlib_extras/Control  Blocks/2nd-Order Filter  FilterType=Lowpass  Fo=750  Zeta=0.707  Initialize=off  Vac_Init=[1 45 60]  Vdc_Init=-0.5  PlotResponse=off  param1=[1 500 1]
      settings: SourceProductName=Simscape Electrical  SourceProductBaseCode=PS
  Demux : Demux  Outputs=3
  Demux1 : Demux  Outputs=3
  Mux : Mux  Inputs=3
  Mux1 : Mux  Inputs=3
  " Vabc*" : Outport
  Iabc* : Outport  Port=2
  " Vdc*" : Outport  Port=3
  wires:
  Mux1/1 -> Iabc*/1
  Demux1/2 -> Mux1/2
  Demux1/3 -> Mux1/3
  "Iabc "/1 -> Demux1/1
  "Vdc "/1 -> " Vdc*"/1
  Mux/1 -> " Vabc*"/1
  Vabc/1 -> Demux/1
  Demux/1 -> Mux/1
  Demux/2 -> Mux/2
  Demux/3 -> Mux/3
  Demux1/1 -> Mux1/1

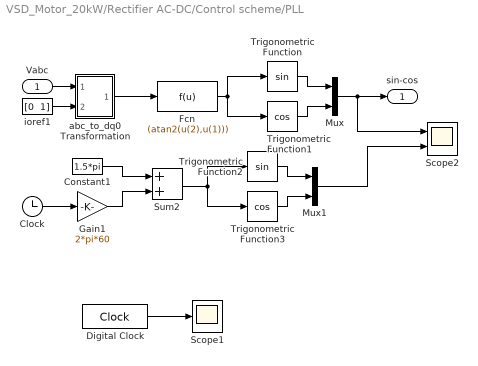
== system VSD_Motor_20kW/Rectifier AC-DC/Control scheme/PLL ==
  Vabc : Inport
  Clock : Clock
  Constant1 : Constant  Value=1.5*pi
  Digital Clock : DigitalClock
  Fcn : Fcn  Expr=(atan2(u(2),u(1)))
  Gain1 : Gain  Gain=2*pi*60
  Mux : Mux  Inputs=2
  Mux1 : Mux  Inputs=2
  Scope1 : Scope
  Scope2 : Scope  NumInputPorts=2
  Sum2 : Sum  SaturateOnIntegerOverflow=on  InputSameDT=on  OutDataTypeStr=Inherit: Same as first input
  Trigonometric Function : Trigonometry
  Trigonometric Function1 : Trigonometry  Operator=cos
  Trigonometric Function2 : Trigonometry
  Trigonometric Function3 : Trigonometry  Operator=cos
  abc_to_dq0 Transformation : Subsystem  mask(abc to dq0 Transformation){}
      mask help:
      | This block performs the  abc to dq0 transformation on a set of three-phase signals. It computes the direct axis Vd, quadratic axis Vq, and zero sequence V0 quantities in a two axis rotating reference frame according to the following transformation:
      |
      | Vd = 2/3*[Va*sin(wt)  + Vb*sin(wt-2pi/3)  +  Vc*sin(wt+2pi/3)]
      | Vq = 2/3*[Va*cos(wt) + Vb*cos(wt-2pi/3) + Vc*cos(wt+2pi/3)]
      | V0 = 1/3*[Va +  Vb  +  Vc ]
      |
      | where w=  rotation speed (rad/s) of the rotating frame.
      |
      | This transformation is commonly used in three-phase electric machine models where it is known as the Park transformation.
      mask Help: web(psbhelp);
  ioref1 : Constant  Value="[0  1]"
  sin-cos : Outport
  wires:
  ioref1/1 -> abc_to_dq0 Transformation/2(sin_cos)
  abc_to_dq0 Transformation/1(dq0) -> Fcn/1
  Fcn/1 -> Trigonometric Function/1, Trigonometric Function1/1
  Trigonometric Function/1 -> Mux/1
  Trigonometric Function1/1 -> Mux/2
  Vabc/1 -> abc_to_dq0 Transformation/1(abc)
  Mux/1 -> sin-cos/1, Scope2/1
  Digital Clock/1 -> Scope1/1
  Clock/1 -> Gain1/1
  Sum2/1 -> Trigonometric Function3/1, Trigonometric Function2/1
  Trigonometric Function2/1 -> Mux1/1
  Trigonometric Function3/1 -> Mux1/2
  Constant1/1 -> Sum2/1
  Gain1/1 -> Sum2/2
  Mux1/1 -> Scope2/2

== system VSD_Motor_20kW/Rectifier AC-DC/Control scheme/SVPWM ==
  note: Subsystem1: calculate the work time of the vector
  note: sector calc: calculate the sector of the reference vector
  Udc : Inport
  Valf : Inport  Port=2
  Vbeta : Inport  Port=3
  Mux1 : Mux  Inputs=2
  Scope1 : Scope  NumInputPorts=2
  Scope2 : Scope
  Scope5 : Scope
  Scope7 : Scope
  T1 : Constant  Value=Ts
  pulse generater : Subsystem
  sector calc : Subsystem
  time calc : Subsystem
  time convert : Subsystem
  time convert1 : Subsystem
  time convert2 : Subsystem
  triangular : simulink/Sources/Repeating Sequence  rep_seq_t=[0 0.5 1]*Ts  rep_seq_y=[0 0.5 0]*Ts
  Out1 : Outport
  wires:
  Mux1/1 -> Scope5/1
  triangular/1 -> pulse generater/4(Tri), Mux1/1, Scope7/1
  time convert2/3(Tcm3) -> pulse generater/3(Tcm3)
  time convert2/2(Tcm2) -> pulse generater/2(Tcm2)
  time convert1/3(Tc) -> time convert2/3(Tc)
  time convert1/2(Tb) -> time convert2/2(Tb)
  time convert1/1(Ta) -> time convert2/1(Ta)
  time convert2/1(Tcm1) -> pulse generater/1(Tcm1), Mux1/2
  time convert/2(t2) -> time convert1/3(t2)
  time convert/1(t1) -> time convert1/2(t1)
  T1/1 -> time calc/2(In2), time convert1/1(Ts)
  sector calc/1(N) -> time convert/4(N), time convert2/4(N), Scope2/1
  time calc/3(Z) -> time convert/3(Z)
  time calc/2(Y) -> time convert/2(Y)
  time calc/1(X) -> time convert/1(X)
  Udc/1 -> time calc/1(In1)
  Vbeta/1 -> sector calc/2(ubeta), time calc/3(In3), Scope1/2
  Valf/1 -> sector calc/1(ualf), Scope1/1, time calc/4(In4)
  pulse generater/1(pulse) -> Out1/1

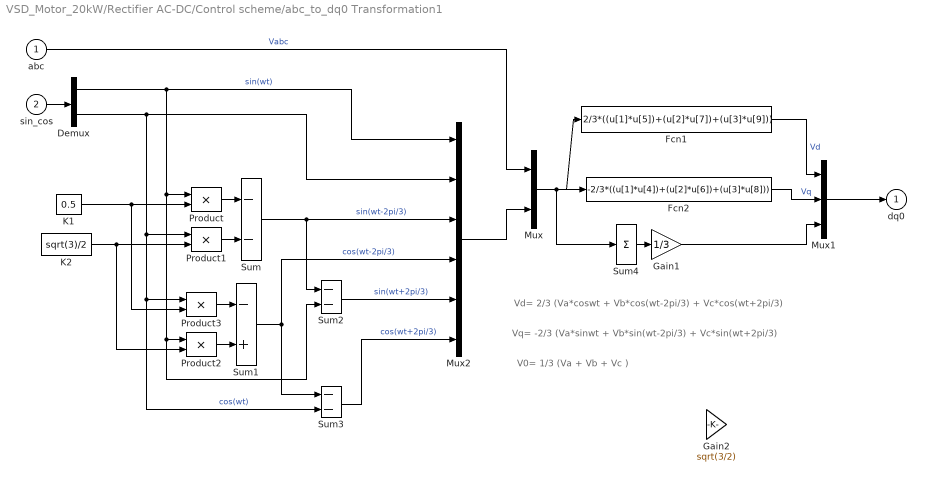
== system VSD_Motor_20kW/Rectifier AC-DC/Control scheme/abc_to_dq0 Transformation1 ==
  note: V0= 1/3 (Va + Vb + Vc )
  note: Vq= -2/3 (Va*sinwt + Vb*sin(wt-2pi/3) + Vc*sin(wt+2pi/3)
  note: Vd= 2/3 (Va*coswt + Vb*cos(wt-2pi/3) + Vc*cos(wt+2pi/3)
  abc : Inport  PortDimensions=3
  sin_cos : Inport  Port=2  PortDimensions=2
  Demux : Demux  Outputs=2
  Fcn1 : Fcn  Expr=2/3*((u[1]*u[5])+(u[2]*u[7])+(u[3]*u[9]))
  Fcn2 : Fcn  Expr=-2/3*((u[1]*u[4])+(u[2]*u[6])+(u[3]*u[8]))
  Gain1 : Gain  Gain=1/3  SaturateOnIntegerOverflow=on  OutDataTypeStr=Inherit: Same as input  ParamDataTypeStr=Inherit: Same as input
  Gain2 : Gain  Gain=sqrt(3/2)  SaturateOnIntegerOverflow=on  OutDataTypeStr=Inherit: Same as input  ParamDataTypeStr=Inherit: Same as input
  K1 : Constant  Value=0.5
  K2 : Constant  Value=sqrt(3)/2
  Mux : Mux  Inputs=2
  Mux1 : Mux  Inputs=3
  Mux2 : Mux  Inputs=6
  Product{,1..3} (4 alike) : Product  SaturateOnIntegerOverflow=on  InputSameDT=on  OutDataTypeStr=Inherit: Same as first input
  Sum : Sum  Inputs=--  SaturateOnIntegerOverflow=on  InputSameDT=on  OutDataTypeStr=Inherit: Same as first input
  Sum1 : Sum  Inputs=-+  SaturateOnIntegerOverflow=on  InputSameDT=on  OutDataTypeStr=Inherit: Same as first input
  Sum2 : Sum  Inputs=--  SaturateOnIntegerOverflow=on  InputSameDT=on  OutDataTypeStr=Inherit: Same as first input
  Sum3 : Sum  Inputs=--  SaturateOnIntegerOverflow=on  InputSameDT=on  OutDataTypeStr=Inherit: Same as first input
  Sum4 : Sum  Inputs=1  SaturateOnIntegerOverflow=on  InputSameDT=on  OutDataTypeStr=Inherit: Same as first input
  dq0 : Outport  InitialOutput=0
  wires:
  Gain1/1 -> Mux1/3
  Fcn1/1 -> Mux1/1  "Vd"
  Mux1/1 -> dq0/1
  Sum4/1 -> Gain1/1
  Mux/1 -> Sum4/1, Fcn1/1, Fcn2/1
  Sum1/1 -> Sum3/1, Mux2/4  "cos(wt-2pi/3)"
  Sum/1 -> Sum2/1, Mux2/3  "sin(wt-2pi/3)"
  K2/1 -> Product2/2, Product1/2
  K1/1 -> Product3/2, Product/2
  Sum2/1 -> Mux2/5  "sin(wt+2pi/3)"
  Sum3/1 -> Mux2/6  "cos(wt+2pi/3)"
  Product2/1 -> Sum1/2
  Product3/1 -> Sum1/1
  Product1/1 -> Sum/2
  Product/1 -> Sum/1
  Demux/1 -> Mux2/1, Sum2/2, Product2/1, Product/1  "sin(wt)"
  Demux/2 -> Mux2/2, Product1/1, Product3/1, Sum3/2  "cos(wt)"
  sin_cos/1 -> Demux/1
  Mux2/1 -> Mux/2
  abc/1 -> Mux/1  "Vabc"
  Fcn2/1 -> Mux1/2  "Vq"

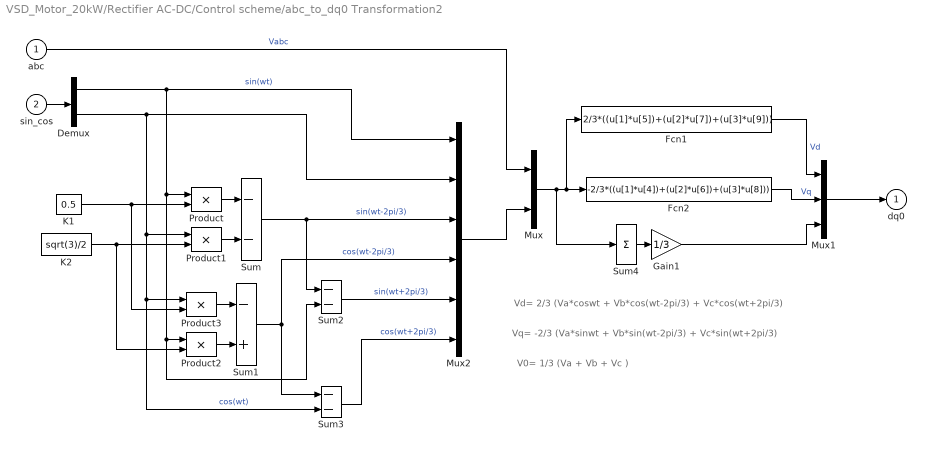
== system VSD_Motor_20kW/Rectifier AC-DC/Control scheme/abc_to_dq0 Transformation2 ==
  note: Vd= 2/3 (Va*coswt + Vb*cos(wt-2pi/3) + Vc*cos(wt+2pi/3)
  note: Vq= -2/3 (Va*sinwt + Vb*sin(wt-2pi/3) + Vc*sin(wt+2pi/3)
  note: V0= 1/3 (Va + Vb + Vc )
  abc : Inport  PortDimensions=3
  sin_cos : Inport  Port=2  PortDimensions=2
  Demux : Demux  Outputs=2
  Fcn1 : Fcn  Expr=2/3*((u[1]*u[5])+(u[2]*u[7])+(u[3]*u[9]))
  Fcn2 : Fcn  Expr=-2/3*((u[1]*u[4])+(u[2]*u[6])+(u[3]*u[8]))
  Gain1 : Gain  Gain=1/3  SaturateOnIntegerOverflow=on  OutDataTypeStr=Inherit: Same as input  ParamDataTypeStr=Inherit: Same as input
  K1 : Constant  Value=0.5
  K2 : Constant  Value=sqrt(3)/2
  Mux : Mux  Inputs=2
  Mux1 : Mux  Inputs=3
  Mux2 : Mux  Inputs=6
  Product{,1..3} (4 alike) : Product  SaturateOnIntegerOverflow=on  InputSameDT=on  OutDataTypeStr=Inherit: Same as first input
  Sum : Sum  Inputs=--  SaturateOnIntegerOverflow=on  InputSameDT=on  OutDataTypeStr=Inherit: Same as first input
  Sum1 : Sum  Inputs=-+  SaturateOnIntegerOverflow=on  InputSameDT=on  OutDataTypeStr=Inherit: Same as first input
  Sum2 : Sum  Inputs=--  SaturateOnIntegerOverflow=on  InputSameDT=on  OutDataTypeStr=Inherit: Same as first input
  Sum3 : Sum  Inputs=--  SaturateOnIntegerOverflow=on  InputSameDT=on  OutDataTypeStr=Inherit: Same as first input
  Sum4 : Sum  Inputs=1  SaturateOnIntegerOverflow=on  InputSameDT=on  OutDataTypeStr=Inherit: Same as first input
  dq0 : Outport  InitialOutput=0
  wires:
  Fcn2/1 -> Mux1/2  "Vq"
  abc/1 -> Mux/1  "Vabc"
  Mux2/1 -> Mux/2
  sin_cos/1 -> Demux/1
  Demux/2 -> Sum3/2, Product3/1, Product1/1, Mux2/2  "cos(wt)"
  Demux/1 -> Product/1, Product2/1, Sum2/2, Mux2/1  "sin(wt)"
  Product/1 -> Sum/1
  Product1/1 -> Sum/2
  Product3/1 -> Sum1/1
  Product2/1 -> Sum1/2
  Sum3/1 -> Mux2/6  "cos(wt+2pi/3)"
  Sum2/1 -> Mux2/5  "sin(wt+2pi/3)"
  K1/1 -> Product/2, Product3/2
  K2/1 -> Product1/2, Product2/2
  Sum/1 -> Mux2/3, Sum2/1  "sin(wt-2pi/3)"
  Sum1/1 -> Mux2/4, Sum3/1  "cos(wt-2pi/3)"
  Mux/1 -> Fcn2/1, Fcn1/1, Sum4/1
  Sum4/1 -> Gain1/1
  Mux1/1 -> dq0/1
  Fcn1/1 -> Mux1/1  "Vd"
  Gain1/1 -> Mux1/3

== system VSD_Motor_20kW/Inverter (DC-AC) and Motor_Controls/SV PWM/SVPWM/pulse generater ==
  Tcm1 : Inport
  Tcm2 : Inport  Port=2
  Tcm3 : Inport  Port=3
  Tri : Inport  Port=4
  Mux : Mux  Inputs=3
  Sum1 : Sum  Inputs=|+-
  Sum2 : Sum  Inputs=|+-
  Sum3 : Sum  Inputs=|+-
  Switch : Switch
  Switch1 : Switch
  Switch2 : Switch
  T : Constant  Value=[0,1]
  T1 : Constant  Value=[1,0]
  pulse : Outport
  wires:
  Tri/1 -> Sum3/1, Sum2/1, Sum1/1
  Sum1/1 -> Switch/2
  Sum2/1 -> Switch1/2
  Sum3/1 -> Switch2/2
  T/1 -> Switch/3, Switch1/3, Switch2/3
  Tcm1/1 -> Sum1/2
  Tcm2/1 -> Sum2/2
  Tcm3/1 -> Sum3/2
  T1/1 -> Switch/1, Switch1/1, Switch2/1
  Switch/1 -> Mux/1
  Switch1/1 -> Mux/2
  Switch2/1 -> Mux/3
  Mux/1 -> pulse/1

== system VSD_Motor_20kW/Inverter (DC-AC) and Motor_Controls/SV PWM/SVPWM/sector calc ==
  ualf : Inport
  ubeta : Inport  Port=2
  Constant : Constant
  Constant1 : Constant  Value=0
  Gain : Gain  Gain=sqrt(3)
  Gain1 : Gain  Gain=-1
  Gain2 : Gain  Gain=4
  Gain3 : Gain  Gain=2
  Saturation : Saturate  UpperLimit=6  LowerLimit=0
  Sum : Sum  Inputs=|+-
  Sum1 : Sum  Inputs=|+-
  Sum2 : Sum  Inputs=|+++
  Switch : Switch
  Switch1 : Switch
  Switch2 : Switch
  N : Outport
  wires:
  Gain/1 -> Gain1/1, Sum1/1
  Gain1/1 -> Sum/1
  ubeta/1 -> Switch/2, Sum/2, Sum1/2
  Constant/1 -> Switch/1, Switch2/1, Switch1/1
  Sum/1 -> Switch1/2
  Sum1/1 -> Switch2/2
  Constant1/1 -> Switch2/3, Switch/3, Switch1/3
  Switch1/1 -> Gain2/1
  Switch2/1 -> Gain3/1
  Switch/1 -> Sum2/1
  Gain2/1 -> Sum2/2
  Gain3/1 -> Sum2/3
  Sum2/1 -> Saturation/1
  ualf/1 -> Gain/1
  Saturation/1 -> N/1

== system VSD_Motor_20kW/Inverter (DC-AC) and Motor_Controls/SV PWM/SVPWM/time calc ==
  In1 : Inport
  In2 : Inport  Port=2
  In3 : Inport  Port=3
  In4 : Inport  Port=4
  Mux : Mux
  ualf1 : Fcn  Expr=sqrt(3)*u(3)*u(2)/u(1)
  ualf2 : Fcn  Expr=(sqrt(3)/2*u(3)+1.5*u(4))*u(2)/u(1)
  ualf3 : Fcn  Expr=(sqrt(3)/2*u(3)-1.5*u(4))*u(2)/u(1)
  X : Outport
  Y : Outport  Port=2
  Z : Outport  Port=3
  wires:
  Mux/1 -> ualf1/1, ualf2/1, ualf3/1
  ualf1/1 -> X/1
  ualf2/1 -> Y/1
  ualf3/1 -> Z/1
  In3/1 -> Mux/3
  In4/1 -> Mux/4
  In1/1 -> Mux/1
  In2/1 -> Mux/2

== system VSD_Motor_20kW/Inverter (DC-AC) and Motor_Controls/SV PWM/SVPWM/time convert ==
  X : Inport
  Y : Inport  Port=2
  Z : Inport  Port=3
  N : Inport  Port=4
  Gain : Gain  Gain=-1
  Gain1 : Gain  Gain=-1
  Gain2 : Gain  Gain=-1
  Multiport Switch1 : MultiPortSwitch  Inputs=6
  Multiport Switch2 : MultiPortSwitch  Inputs=6
  t1 : Outport
  t2 : Outport  Port=2
  wires:
  N/1 -> Multiport Switch1/1, Multiport Switch2/1
  X/1 -> Multiport Switch2/6, Multiport Switch1/4, Gain/1
  Y/1 -> Multiport Switch2/3, Multiport Switch1/2, Gain1/1
  Z/1 -> Multiport Switch1/5, Multiport Switch2/2, Gain2/1
  Gain/1 -> Multiport Switch1/3, Multiport Switch2/5
  Gain2/1 -> Multiport Switch2/4, Multiport Switch1/7
  Gain1/1 -> Multiport Switch1/6, Multiport Switch2/7
  Multiport Switch2/1 -> t1/1
  Multiport Switch1/1 -> t2/1

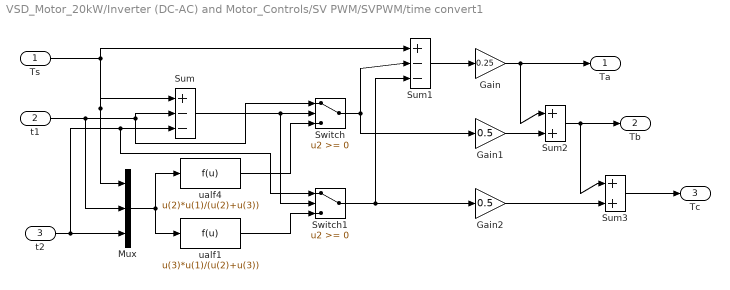
== system VSD_Motor_20kW/Inverter (DC-AC) and Motor_Controls/SV PWM/SVPWM/time convert1 ==
  Ts : Inport
  t1 : Inport  Port=2
  t2 : Inport  Port=3
  Gain : Gain  Gain=0.25
  Gain1 : Gain  Gain=0.5
  Gain2 : Gain  Gain=0.5
  Mux : Mux  Inputs=3
  Sum : Sum  Inputs=|+--
  Sum1 : Sum  Inputs=|+--
  Sum2 : Sum  Inputs=|++
  Sum3 : Sum  Inputs=|++
  Switch : Switch
  Switch1 : Switch
  ualf1 : Fcn  Expr=u(3)*u(1)/(u(2)+u(3))
  ualf4 : Fcn  Expr=u(2)*u(1)/(u(2)+u(3))
  Ta : Outport
  Tb : Outport  Port=2
  Tc : Outport  Port=3
  wires:
  t1/1 -> Switch/1, Sum/2, Mux/2
  t2/1 -> Switch1/1, Sum/3, Mux/3
  Mux/1 -> ualf4/1, ualf1/1
  Sum/1 -> Switch/2, Switch1/2
  ualf4/1 -> Switch/3
  ualf1/1 -> Switch1/3
  Switch/1 -> Sum1/2, Gain1/1
  Ts/1 -> Sum1/1, Mux/1, Sum/1
  Switch1/1 -> Sum1/3, Gain2/1
  Sum1/1 -> Gain/1
  Gain/1 -> Ta/1, Sum2/1
  Gain1/1 -> Sum2/2
  Sum2/1 -> Tb/1, Sum3/1
  Gain2/1 -> Sum3/2
  Sum3/1 -> Tc/1

== system VSD_Motor_20kW/Inverter (DC-AC) and Motor_Controls/SV PWM/SVPWM/time convert2 ==
  Ta : Inport
  Tb : Inport  Port=2
  Tc : Inport  Port=3
  N : Inport  Port=4
  Multiport Switch1 : MultiPortSwitch  Inputs=6
  Multiport Switch2 : MultiPortSwitch  Inputs=6
  Multiport Switch3 : MultiPortSwitch  Inputs=6
  Tcm1 : Outport
  Tcm2 : Outport  Port=2
  Tcm3 : Outport  Port=3
  wires:
  Tb/1 -> Multiport Switch2/7, Multiport Switch2/2, Multiport Switch3/6, Multiport Switch3/3, Multiport Switch1/5, Multiport Switch1/4
  Ta/1 -> Multiport Switch3/7, Multiport Switch3/5, Multiport Switch1/6, Multiport Switch1/2, Multiport Switch2/4, Multiport Switch2/3
  Tc/1 -> Multiport Switch2/6, Multiport Switch2/5, Multiport Switch1/7, Multiport Switch3/4, Multiport Switch3/2, Multiport Switch1/3
  Multiport Switch2/1 -> Tcm1/1
  Multiport Switch1/1 -> Tcm2/1
  Multiport Switch3/1 -> Tcm3/1
  N/1 -> Multiport Switch3/1, Multiport Switch2/1, Multiport Switch1/1

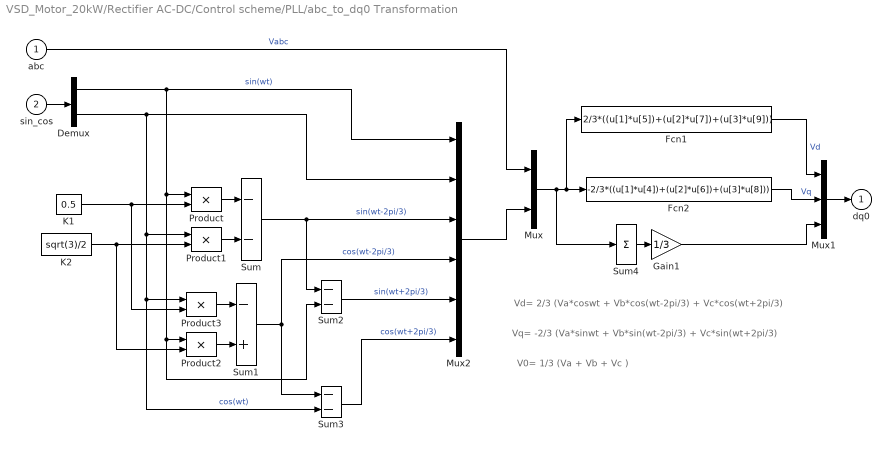
== system VSD_Motor_20kW/Rectifier AC-DC/Control scheme/PLL/abc_to_dq0 Transformation ==
  note: V0= 1/3 (Va + Vb + Vc )
  note: Vq= -2/3 (Va*sinwt + Vb*sin(wt-2pi/3) + Vc*sin(wt+2pi/3)
  note: Vd= 2/3 (Va*coswt + Vb*cos(wt-2pi/3) + Vc*cos(wt+2pi/3)
  abc : Inport  PortDimensions=3
  sin_cos : Inport  Port=2  PortDimensions=2
  Demux : Demux  Outputs=2
  Fcn1 : Fcn  Expr=2/3*((u[1]*u[5])+(u[2]*u[7])+(u[3]*u[9]))
  Fcn2 : Fcn  Expr=-2/3*((u[1]*u[4])+(u[2]*u[6])+(u[3]*u[8]))
  Gain1 : Gain  Gain=1/3  SaturateOnIntegerOverflow=on  OutDataTypeStr=Inherit: Same as input  ParamDataTypeStr=Inherit: Same as input
  K1 : Constant  Value=0.5
  K2 : Constant  Value=sqrt(3)/2
  Mux : Mux  Inputs=2
  Mux1 : Mux  Inputs=3
  Mux2 : Mux  Inputs=6
  Product{,1..3} (4 alike) : Product  SaturateOnIntegerOverflow=on  InputSameDT=on  OutDataTypeStr=Inherit: Same as first input
  Sum : Sum  Inputs=--  SaturateOnIntegerOverflow=on  InputSameDT=on  OutDataTypeStr=Inherit: Same as first input
  Sum1 : Sum  Inputs=-+  SaturateOnIntegerOverflow=on  InputSameDT=on  OutDataTypeStr=Inherit: Same as first input
  Sum2 : Sum  Inputs=--  SaturateOnIntegerOverflow=on  InputSameDT=on  OutDataTypeStr=Inherit: Same as first input
  Sum3 : Sum  Inputs=--  SaturateOnIntegerOverflow=on  InputSameDT=on  OutDataTypeStr=Inherit: Same as first input
  Sum4 : Sum  Inputs=1  SaturateOnIntegerOverflow=on  InputSameDT=on  OutDataTypeStr=Inherit: Same as first input
  dq0 : Outport  InitialOutput=0
  wires:
  Gain1/1 -> Mux1/3
  Fcn1/1 -> Mux1/1  "Vd"
  Mux1/1 -> dq0/1
  Sum4/1 -> Gain1/1
  Mux/1 -> Fcn1/1, Fcn2/1, Sum4/1
  Sum1/1 -> Sum3/1, Mux2/4  "cos(wt-2pi/3)"
  Sum/1 -> Sum2/1, Mux2/3  "sin(wt-2pi/3)"
  K2/1 -> Product2/2, Product1/2
  K1/1 -> Product3/2, Product/2
  Sum2/1 -> Mux2/5  "sin(wt+2pi/3)"
  Sum3/1 -> Mux2/6  "cos(wt+2pi/3)"
  Product2/1 -> Sum1/2
  Product3/1 -> Sum1/1
  Product1/1 -> Sum/2
  Product/1 -> Sum/1
  Demux/1 -> Mux2/1, Sum2/2, Product2/1, Product/1  "sin(wt)"
  Demux/2 -> Mux2/2, Product1/1, Product3/1, Sum3/2  "cos(wt)"
  sin_cos/1 -> Demux/1
  Mux2/1 -> Mux/2
  abc/1 -> Mux/1  "Vabc"
  Fcn2/1 -> Mux1/2  "Vq"

== system VSD_Motor_20kW/Rectifier AC-DC/Control scheme/SVPWM/pulse generater ==
  Tcm1 : Inport
  Tcm2 : Inport  Port=2
  Tcm3 : Inport  Port=3
  Tri : Inport  Port=4
  Mux : Mux  Inputs=3
  Sum1 : Sum  Inputs=|+-
  Sum2 : Sum  Inputs=|+-
  Sum3 : Sum  Inputs=|+-
  Switch : Switch
  Switch1 : Switch
  Switch2 : Switch
  T : Constant  Value=[0,1]
  T1 : Constant  Value=[1,0]
  pulse : Outport
  wires:
  Tri/1 -> Sum3/1, Sum2/1, Sum1/1
  Sum1/1 -> Switch/2
  Sum2/1 -> Switch1/2
  Sum3/1 -> Switch2/2
  T/1 -> Switch/3, Switch1/3, Switch2/3
  Tcm1/1 -> Sum1/2
  Tcm2/1 -> Sum2/2
  Tcm3/1 -> Sum3/2
  T1/1 -> Switch/1, Switch1/1, Switch2/1
  Switch/1 -> Mux/1
  Switch1/1 -> Mux/2
  Switch2/1 -> Mux/3
  Mux/1 -> pulse/1

== system VSD_Motor_20kW/Rectifier AC-DC/Control scheme/SVPWM/sector calc ==
  ualf : Inport
  ubeta : Inport  Port=2
  Constant : Constant
  Constant1 : Constant  Value=0
  Gain : Gain  Gain=sqrt(3)
  Gain1 : Gain  Gain=-1
  Gain2 : Gain  Gain=4
  Gain3 : Gain  Gain=2
  Saturation : Saturate  UpperLimit=6  LowerLimit=0
  Sum : Sum  Inputs=|+-
  Sum1 : Sum  Inputs=|+-
  Sum2 : Sum  Inputs=|+++
  Switch : Switch
  Switch1 : Switch
  Switch2 : Switch
  N : Outport
  wires:
  Gain/1 -> Gain1/1, Sum1/1
  Gain1/1 -> Sum/1
  ubeta/1 -> Switch/2, Sum/2, Sum1/2
  Constant/1 -> Switch/1, Switch2/1, Switch1/1
  Sum/1 -> Switch1/2
  Sum1/1 -> Switch2/2
  Constant1/1 -> Switch2/3, Switch/3, Switch1/3
  Switch1/1 -> Gain2/1
  Switch2/1 -> Gain3/1
  Switch/1 -> Sum2/1
  Gain2/1 -> Sum2/2
  Gain3/1 -> Sum2/3
  Sum2/1 -> Saturation/1
  ualf/1 -> Gain/1
  Saturation/1 -> N/1

== system VSD_Motor_20kW/Rectifier AC-DC/Control scheme/SVPWM/time calc ==
  In1 : Inport
  In2 : Inport  Port=2
  In3 : Inport  Port=3
  In4 : Inport  Port=4
  Mux : Mux
  ualf1 : Fcn  Expr=sqrt(3)*u(3)*u(2)/u(1)
  ualf2 : Fcn  Expr=(sqrt(3)/2*u(3)+1.5*u(4))*u(2)/u(1)
  ualf3 : Fcn  Expr=(sqrt(3)/2*u(3)-1.5*u(4))*u(2)/u(1)
  X : Outport
  Y : Outport  Port=2
  Z : Outport  Port=3
  wires:
  Mux/1 -> ualf1/1, ualf2/1, ualf3/1
  ualf1/1 -> X/1
  ualf2/1 -> Y/1
  ualf3/1 -> Z/1
  In3/1 -> Mux/3
  In4/1 -> Mux/4
  In1/1 -> Mux/1
  In2/1 -> Mux/2

== system VSD_Motor_20kW/Rectifier AC-DC/Control scheme/SVPWM/time convert ==
  X : Inport
  Y : Inport  Port=2
  Z : Inport  Port=3
  N : Inport  Port=4
  Gain : Gain  Gain=-1
  Gain1 : Gain  Gain=-1
  Gain2 : Gain  Gain=-1
  Multiport Switch1 : MultiPortSwitch  Inputs=6
  Multiport Switch2 : MultiPortSwitch  Inputs=6
  t1 : Outport
  t2 : Outport  Port=2
  wires:
  N/1 -> Multiport Switch1/1, Multiport Switch2/1
  X/1 -> Multiport Switch2/6, Multiport Switch1/4, Gain/1
  Y/1 -> Multiport Switch2/3, Multiport Switch1/2, Gain1/1
  Z/1 -> Multiport Switch1/5, Multiport Switch2/2, Gain2/1
  Gain/1 -> Multiport Switch1/3, Multiport Switch2/5
  Gain2/1 -> Multiport Switch2/4, Multiport Switch1/7
  Gain1/1 -> Multiport Switch1/6, Multiport Switch2/7
  Multiport Switch2/1 -> t1/1
  Multiport Switch1/1 -> t2/1

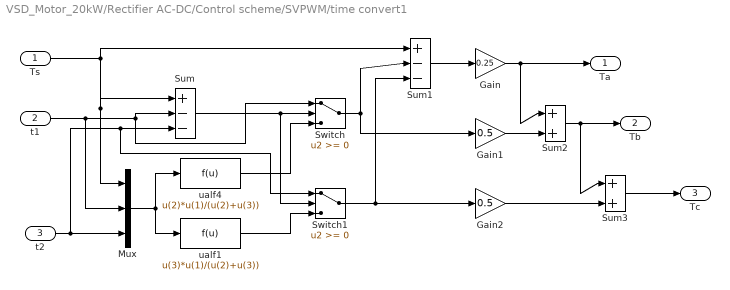
== system VSD_Motor_20kW/Rectifier AC-DC/Control scheme/SVPWM/time convert1 ==
  Ts : Inport
  t1 : Inport  Port=2
  t2 : Inport  Port=3
  Gain : Gain  Gain=0.25
  Gain1 : Gain  Gain=0.5
  Gain2 : Gain  Gain=0.5
  Mux : Mux  Inputs=3
  Sum : Sum  Inputs=|+--
  Sum1 : Sum  Inputs=|+--
  Sum2 : Sum  Inputs=|++
  Sum3 : Sum  Inputs=|++
  Switch : Switch
  Switch1 : Switch
  ualf1 : Fcn  Expr=u(3)*u(1)/(u(2)+u(3))
  ualf4 : Fcn  Expr=u(2)*u(1)/(u(2)+u(3))
  Ta : Outport
  Tb : Outport  Port=2
  Tc : Outport  Port=3
  wires:
  t1/1 -> Switch/1, Sum/2, Mux/2
  t2/1 -> Switch1/1, Sum/3, Mux/3
  Mux/1 -> ualf4/1, ualf1/1
  Sum/1 -> Switch/2, Switch1/2
  ualf4/1 -> Switch/3
  ualf1/1 -> Switch1/3
  Switch/1 -> Sum1/2, Gain1/1
  Ts/1 -> Sum1/1, Mux/1, Sum/1
  Switch1/1 -> Sum1/3, Gain2/1
  Sum1/1 -> Gain/1
  Gain/1 -> Ta/1, Sum2/1
  Gain1/1 -> Sum2/2
  Sum2/1 -> Tb/1, Sum3/1
  Gain2/1 -> Sum3/2
  Sum3/1 -> Tc/1
